simulink library "mylib1"  (R2021a)
settings: Solver=VariableStepAuto  StartTime=0.0  StopTime=10.0  RelTol=1e-3
undefined symbols (not defined in the file or in its folder): magnitude
settings Model: Creator=Aula  LastModifiedBy=Aula

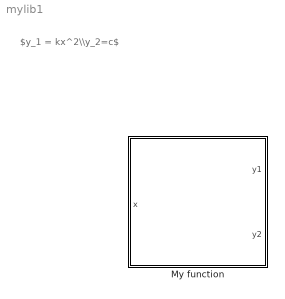
== system mylib1 ==
  note: $y_1 = kx^2\\y_2=c$
  My function : Subsystem  mask(Função Matemática){k=1, c=0}
      mask prompts: k "Ganho (k)"; c "Constante (c)"
      mask help: Realiza a operação para obter y1 e y2
      mask init:
      | disp('y1 = kx^2; y2 = c');
      mask Help:
      | ganho k
      | constante c
      | entrada x
      | saidas y1 e y2

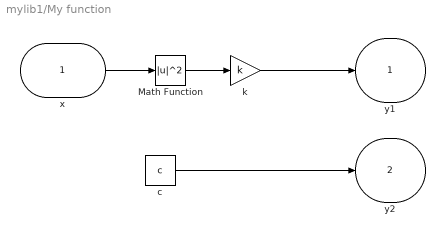
== system mylib1/My function ==
  x : Inport
  Math Function : Math  Operator=magnitude^2  SaturateOnIntegerOverflow=on
  c : Constant  Value=c
  k : Gain  Gain=k
  y1 : Outport
  y2 : Outport  Port=2
  wires:
  c/1 -> y2/1
  Math Function/1 -> k/1
  x/1 -> Math Function/1
  k/1 -> y1/1
